simulink model "model_all"  (R2017b)
settings: Solver=ode45  StartTime=0.0  StopTime=10.0  RelTol=1e-3  EnableMultiTasking=on
values from neighbouring files (symbols this model uses):
  a = moment(pwm==0)    [Helicopter_main.m]    (also in Helicopter_main_test.m = moment(pwm==0)/-sin(-0.5223); Lin_simulink.mat = -0.153036; Lin_simulink_test.mat = -0.153036; parametry.m = 0)
  alpha_0 = -28.13    [Helicopter_main.m]    (also in Helicopter_main_test.m = parameters(3); Lin_simulink.mat = -0.522258237308; Lin_simulink_test.mat = -0.52225830565)
  f_h = 1e-4    (= 0.0001)    [Helicopter_main.m]    (also in Helicopter_main_test.m = decision(1); parametry.m = 0)
  f_v = 0    [Helicopter_main.m]    (also in Helicopter_main_test.m = parameters(2); parametry.m)
  I_v = lsqnonlin(cel, I_v, 0,[],options)    [Helicopter_main.m]    (also in Helicopter_main_test.m; parametry.m = 0)
  Ih = lsqnonlin(cel, Ih, 0,[],options)    [Helicopter_main.m]    (also in parametry.m = 0)
  J_h = 0    [parametry.m]
  J_v = 0    [Helicopter_main.m]    (also in Helicopter_main_test.m = parameters(1); parametry.m)
  lh = 0    [parametry.m]
  wsp_M_V = polyfit(v/60, moment, 5)    [Helicopter_main.m]    (also in Helicopter_main_test.m = polyfit(v, moment, 5); Lin_simulink.mat = [-2.46242484187e-10 4.61213078344e-09 2.0169387865e-06 1.989; Lin_simulink_test.mat = [-2.51456949125e-14 2.95925329869e-12 8.13117134031e-09 5.04)
  wsp_U_V = polyfit(pred,PWM,5)    [Helicopter_main.m]    (also in Helicopter_main_test.m; Lin_simulink.mat = [-7.28749420126e-10 2.12446681505e-08 6.5068856079e-06 -2.60; Lin_simulink_test.mat = [-7.44181518745e-14 1.363108664e-11 2.62321306545e-08 -6.605)
undefined symbols (not defined in the file or in its folder): Fh, Hh, uh, uv
libraries: simulink x1
settings Model: Creator=Student  LastModifiedBy=Marcin
settings DataIOCC: LimitDataPoints=on  SaveFormat=Array
settings OptimizationCC: LifeSpan=inf
settings DebuggingCC: SFUnexpectedBacktrackingDiag=warning  SFNoUnconditionalDefaultTransitionDiag=warning  SFExecutionAtInitializationDiag=none
settings HardwareCC: ProdBitPerPointer=32  ProdBitPerSizeT=32  ProdBitPerPtrDiffT=32  ProdLargestAtomicFloat=None  ProdIntDivRoundTo=Undefined  ProdEndianess=Unspecified  ProdWordSize=32  ProdHWDeviceType=32-bit Generic
settings ModelReferenceCC: PropagateSignalLabelsOutOfModel=off
settings CodeAppCC: StateflowObjectComments=on
settings GRTTargetCC: TargetLangStandard=C89/C90 (ANSI)  GeneratePreprocessorConditionals=Disable all
settings ConfigComp: CovMetricSettings=dw  CovHtmlReporting=on  CovSaveCumulativeToWorkspaceVar=on  CovSaveSingleToWorkspaceVar=on  CovExternalEMLEnable=off

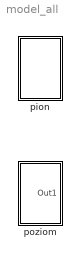
== system model_all ==
  "pion " : Subsystem
  poziom : Subsystem

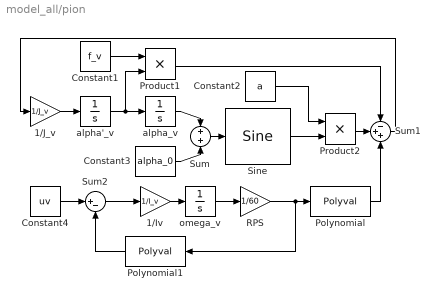
== system model_all/pion  ==
  1/Iv : Gain  Gain=1/I_v
  1/J_v : Gain  Gain=1/J_v
  Constant1 : Constant  Value=f_v
  Constant2 : Constant  Value=a
  Constant3 : Constant  Value=alpha_0
  Constant4 : Constant  Value=uv
  Polynomial : Polyval  Coefs=wsp_M_V
  Polynomial1 : Polyval  Coefs=wsp_U_V
  Product1 : Product
  Product2 : Product
  RPS : Gain  Gain=1/60
  Sine : simulink/Lookup Tables/Sine  Formula=sin(2*pi*u)  NumDataPoints=(2^5)+1  OutputWordLength=16  InternalRulePriority=Speed
      settings: SourceProductName=Simulink
  Sum : Sum  Inputs=+|+
  Sum1 : Sum  Inputs=-++
  Sum2 : Sum  Inputs=|+-
  alpha'_v : Integrator
  alpha_v : Integrator
  omega_v : Integrator
  wires:
  alpha'_v/1 -> Product1/2, alpha_v/1
  1/J_v/1 -> alpha'_v/1
  Sine/1 -> Product2/2
  Product2/1 -> Sum1/2
  Sum1/1 -> 1/J_v/1
  Product1/1 -> Sum1/1
  Sum/1 -> Sine/1
  alpha_v/1 -> Sum/1
  1/Iv/1 -> omega_v/1
  Constant1/1 -> Product1/1
  Constant3/1 -> Sum/2
  Polynomial/1 -> Sum1/3
  omega_v/1 -> RPS/1
  Constant2/1 -> Product2/1
  Sum2/1 -> 1/Iv/1
  Constant4/1 -> Sum2/1
  Polynomial1/1 -> Sum2/2
  RPS/1 -> Polynomial1/1, Polynomial/1

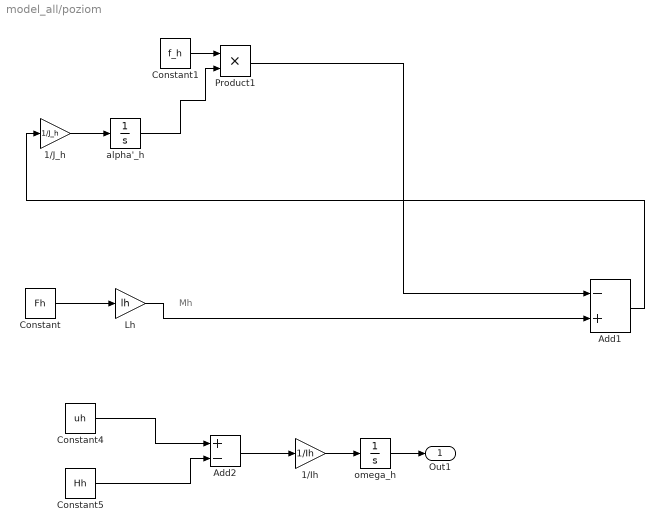
== system model_all/poziom ==
  note: Mh
  1/Ih : Gain  Gain=1/Ih
  1/J_h : Gain  Gain=1/J_h
  Add1 : Sum  Inputs=-+
  Add2 : Sum  Inputs=+-
  Constant : Constant  Value=Fh
  Constant1 : Constant  Value=f_h
  Constant4 : Constant  Value=uh
  Constant5 : Constant  Value=Hh
  Lh : Gain  Gain=lh
  Product1 : Product
  alpha'_h : Integrator
  omega_h : Integrator
  Out1 : Outport
  wires:
  alpha'_h/1 -> Product1/2
  1/J_h/1 -> alpha'_h/1
  Add1/1 -> 1/J_h/1
  Product1/1 -> Add1/1
  Constant/1 -> Lh/1
  Add2/1 -> 1/Ih/1
  1/Ih/1 -> omega_h/1
  Constant1/1 -> Product1/1
  Constant4/1 -> Add2/1
  Lh/1 -> Add1/2
  omega_h/1 -> Out1/1
  Constant5/1 -> Add2/2
